simulink model "test3"  (R2019a)
settings: Solver=VariableStepAuto  StartTime=0.0  StopTime=10  RelTol=1e-3
settings Model: Creator=dell  LastModifiedBy=dell

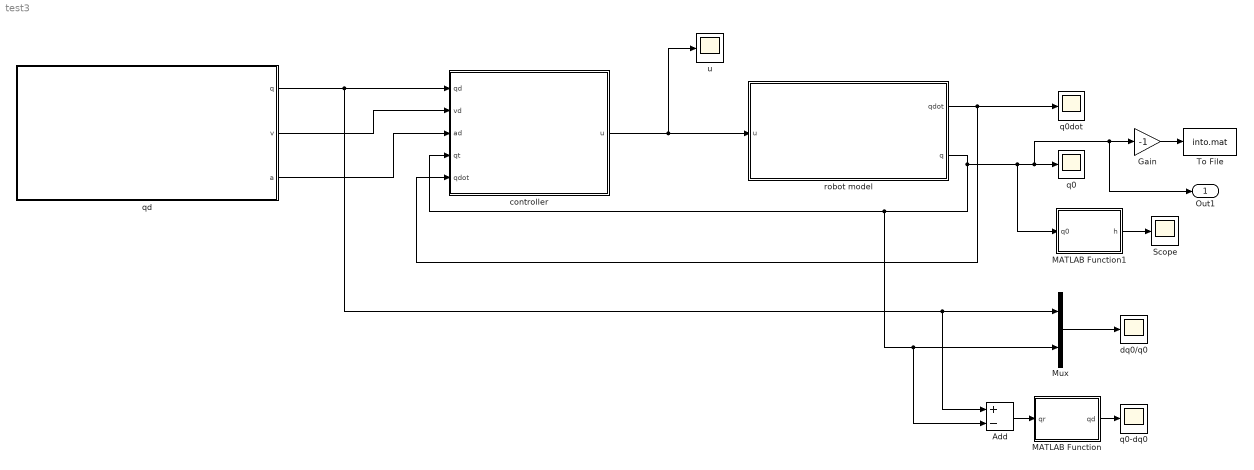
== system test3 ==
  Add : Sum  Inputs=+-
  Gain : Gain  Gain=-1
  MATLAB Function : MATLAB Function  TreatAsAtomicUnit=on
  MATLAB Function1 : MATLAB Function  TreatAsAtomicUnit=on
  Mux : Mux  Inputs=2
  Scope : Scope
  To File : ToFile  Filename=into.mat  SaveFormat=Timeseries
  controller : Subsystem
  dq0/q0 : Scope
  q0 : Scope
  q0-dq0 : Scope
  q0dot : Scope
  qd : Subsystem
  robot model : Subsystem
  u : Scope
  Out1 : Outport
  wires:
  Add/1 -> MATLAB Function/1(qr)
  qd/3("a ") -> controller/3(ad)
  controller/1("u ") -> u/1, robot model/1(u)
  robot model/1(qdot) -> q0dot/1, controller/5(qdot)
  Mux/1 -> dq0/q0/1
  qd/1(q) -> Add/1, Mux/1, controller/1(qd)
  qd/2(v) -> controller/2(vd)
  MATLAB Function/1(qd) -> q0-dq0/1
  MATLAB Function1/1(h) -> Scope/1
  Gain/1 -> To File/1
  robot model/2("q ") -> Add/2, Mux/2, controller/4(qt), MATLAB Function1/1(q0), Out1/1, Gain/1, q0/1

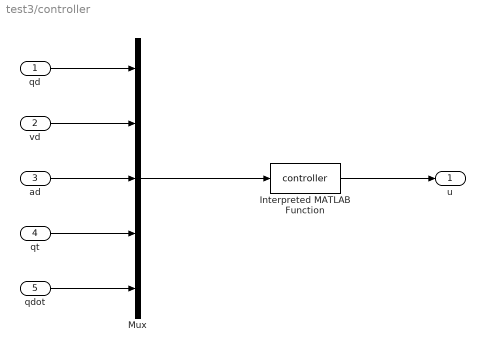
== system test3/controller ==
  qd : Inport
  vd : Inport  Port=2
  ad : Inport  Port=3
  qt : Inport  Port=4
  qdot : Inport  Port=5
  Interpreted MATLAB Function : MATLABFcn  MATLABFcn=controller
  Mux : Mux  Inputs=5
  "u " : Outport
  wires:
  Mux/1 -> Interpreted MATLAB Function/1
  qd/1 -> Mux/1
  Interpreted MATLAB Function/1 -> "u "/1
  vd/1 -> Mux/2
  ad/1 -> Mux/3
  qt/1 -> Mux/4
  qdot/1 -> Mux/5

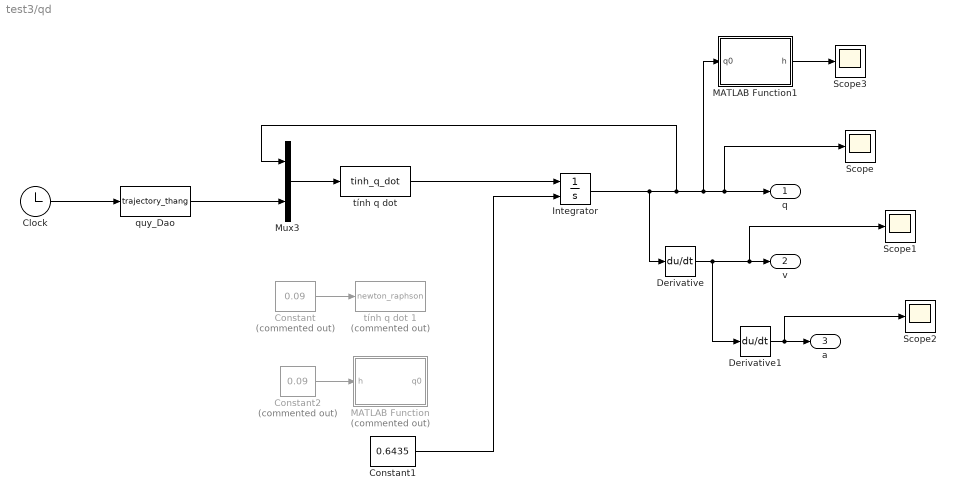
== system test3/qd ==
  Clock : Clock
  Constant : Constant  Commented=on  Value=0.09
  Constant1 : Constant  Value=0.6435
  Constant2 : Constant  Commented=on  Value=0.09
  Derivative : Derivative
  Derivative1 : Derivative
  Integrator : Integrator  InitialConditionSource=external
  MATLAB Function : MATLAB Function  Commented=on  TreatAsAtomicUnit=on
  MATLAB Function1 : MATLAB Function  TreatAsAtomicUnit=on
  Mux3 : Mux  Inputs=2
  Scope{,1..3} (4 alike) : Scope
  quy_Dao : MATLABFcn  MATLABFcn=trajectory_thang  OutputDimensions=2
  "tính q dot " : MATLABFcn  MATLABFcn=tinh_q_dot  OutputDimensions=1
  tính q dot 1 : MATLABFcn  Commented=on  MATLABFcn=newton_raphson  OutputDimensions=1
  q : Outport
  v : Outport  Port=2
  "a " : Outport  Port=3
  wires:
  Clock/1 -> quy_Dao/1
  "tính q dot "/1 -> Integrator/1
  Integrator/1 -> Derivative/1, Mux3/1, MATLAB Function1/1(q0), Scope/1, q/1
  quy_Dao/1 -> Mux3/2
  Mux3/1 -> "tính q dot "/1
  Derivative/1 -> Scope1/1, v/1, Derivative1/1
  Derivative1/1 -> Scope2/1, "a "/1
  MATLAB Function1/1(h) -> Scope3/1
  Constant/1 -> tính q dot 1/1
  Constant2/1 -> MATLAB Function/1(h)
  Constant1/1 -> Integrator/2

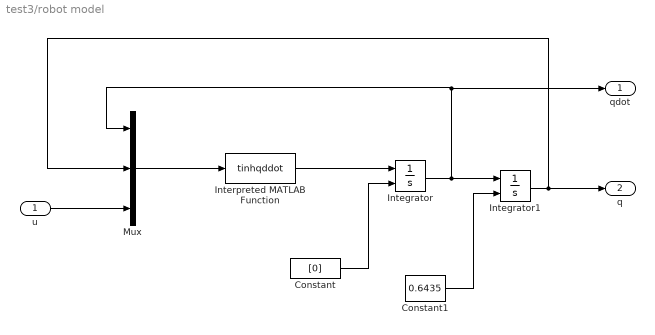
== system test3/robot model ==
  u : Inport
  Constant : Constant  Value=[0]
  Constant1 : Constant  Value=0.6435
  Integrator : Integrator  InitialConditionSource=external
  Integrator1 : Integrator  InitialConditionSource=external
  Interpreted MATLAB Function : MATLABFcn  MATLABFcn=tinhqddot
  Mux : Mux  Inputs=3
  qdot : Outport
  "q " : Outport  Port=2
  wires:
  Mux/1 -> Interpreted MATLAB Function/1
  Integrator/1 -> Mux/1, qdot/1, Integrator1/1
  u/1 -> Mux/3
  Integrator1/1 -> Mux/2, "q "/1
  Interpreted MATLAB Function/1 -> Integrator/1
  Constant/1 -> Integrator/2
  Constant1/1 -> Integrator1/2

== matlab function test3/qd/MATLAB Function1 ==
  data: q0 input; h output
function h = fcn(q0)
a=0.075;
h=2*a*sin(q0);

== matlab function test3/qd/MATLAB Function ==
  data: h input; q0 output
function q0 = fcn(h)
 a=0.075;
q0=asin(h/2*a);
%q0=q1*pi/180;

== matlab function test3/MATLAB Function1 ==
  data: q0 input; h output
function h = fcn(q0)
a=0.075;
h=2*a*sin(q0);

== matlab function test3/MATLAB Function ==
  data: qr input; qd output
function qd = fcn(qr)
qd=qr*180/pi;
